simulink model "SecRwLtStHdrstUpwdDnwdHolderChk"  (R2018b)
settings: Solver=FixedStepDiscrete  StartTime=0.0  StopTime=10.0  FixedStep=0.01  RelTol=1e-3
libraries: simulink x1
settings Model: Creator=sn2xws  LastModifiedBy=sn2xws
settings Model: ModifiedHistory=|
  | 2023/11/7
  | V2.3.0 Bug555749  童锁需要停止md21 22 25 26
settings DataIOCC: SaveFormat=StructureWithTime
settings OptimizationCC: DefaultParameterBehavior=Inlined  EnhancedBackFolding=on  PassReuseOutputArgsAs=Individual arguments  ZeroExternalMemoryAtStartup=off  ZeroInternalMemoryAtStartup=off  OptimizeBlockOrder=speed  DifferentSizesBufferReuse=on  OptimizationCustomize=off
settings DebuggingCC: ParameterTunabilityLossMsg=error
settings ModelReferenceCC: ModelReferenceNumInstancesAllowed=Single
settings SFSimCC: MATLABDynamicMemAlloc=off
settings RTWCC: SystemTargetFile=autosar.tlc  GenCodeOnly=on  TemplateMakefile=ert_default_tmf  Description=AUTOSAR  GenerateReport=on  IncludeHyperlinkInReport=on  LaunchReport=on  GenerateTraceInfo=on  GenerateTraceReport=on  GenerateTraceReportSl=on  GenerateTraceReportSf=on  GenerateTraceReportEml=on
settings CodeAppCC: ForceParamTrailComments=on  IgnoreCustomStorageClasses=off  OperatorAnnotations=on  SimulinkDataObjDesc=on  SFDataObjDesc=on  InsertBlockDesc=on
settings STFCustomTargetCC: TargetLangStandard=C99 (ISO)  MultiwordLength=256  ParMdlRefBuildCompliant=on  CompOptLevelCompliant=on  IncludeMdlTerminateFcn=off  CombineOutputUpdateFcns=on  SuppressErrorStatus=on  ERTCustomFileBanners=on  SupportNonFinite=off  SupportComplex=off  SupportContinuousTime=off  SupportNonInlinedSFcns=off  RemoveResetFunc=on  MATLABClassNameForMDSCustomization=Simulink.SoftwareTarget.ERTCustomization  AutosarCompliant=on  UseToolchainInfoCompliant=on  LookupTableObjectStructAxisOrder=2,1,3,4,...  LUTObjectStructOrderEvenSpacing=Size,Table,Breakpoints  SystemTargetFile=autosar.tlc
settings ERTTargetCC: TargetLangStandard=C99 (ISO)  ConcurrentExecutionCompliant=off  IncludeMdlTerminateFcn=off  SuppressErrorStatus=on  SupportNonFinite=off  SupportComplex=off  ModelStepFunctionPrototypeControlCompliant=off  CPPClassGenCompliant=off  AutosarCompliant=on  LookupTableObjectStructAxisOrder=2,1,3,4,...  LUTObjectStructOrderEvenSpacing=Size,Table,Breakpoints  InlinedParameterPlacement=NonHierarchical  ERTCustomFileTemplate=example_file_process.tlc  ERTFilePackagingFormat=Compact

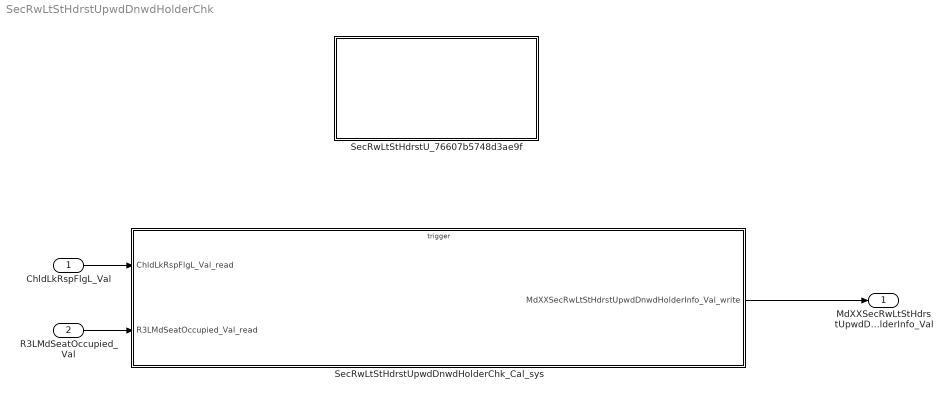
== system SecRwLtStHdrstUpwdDnwdHolderChk ==
  ChldLkRspFlgL_Val : Inport  OutDataTypeStr=boolean  PortDimensions=1
  R3LMdSeatOccupied_Val : Inport  Port=2  OutDataTypeStr=boolean  PortDimensions=1
  SecRwLtStHdrstU_76607b5748d3ae9f : Subsystem
  SecRwLtStHdrstUpwdDnwdHolderChk_Cal_sys : Subsystem
  MdXXSecRwLtStHdrstUpwdDnwdHolderInfo_Val : Outport  OutDataTypeStr=uint32  PortDimensions=1
  wires:
  ChldLkRspFlgL_Val/1 -> SecRwLtStHdrstUpwdDnwdHolderChk_Cal_sys/1(ChldLkRspFlgL_Val_read)
  R3LMdSeatOccupied_Val/1 -> SecRwLtStHdrstUpwdDnwdHolderChk_Cal_sys/2(R3LMdSeatOccupied_Val_read)
  SecRwLtStHdrstUpwdDnwdHolderChk_Cal_sys/1(MdXXSecRwLtStHdrstUpwdDnwdHolderInfo_Val_write) -> MdXXSecRwLtStHdrstUpwdDnwdHolderInfo_Val/1

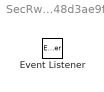
== system SecRwLtStHdrstUpwdDnwdHolderChk/SecRwLtStHdrstU_76607b5748d3ae9f ==
  Event Listener : EventListener  EventName=reset

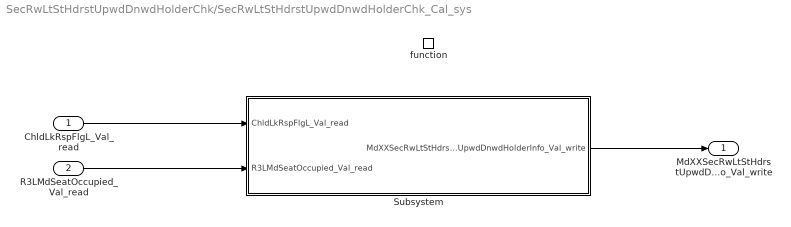
== system SecRwLtStHdrstUpwdDnwdHolderChk/SecRwLtStHdrstUpwdDnwdHolderChk_Cal_sys ==
  ChldLkRspFlgL_Val_read : Inport
  R3LMdSeatOccupied_Val_read : Inport  Port=2
  function : TriggerPort  TriggerType=function-call  IsSimulinkFunction=on  FunctionName=SecRwLtStHdrstUpwdDnwdHolderChk_Cal  VariantControl=(inherit)
  Subsystem : Subsystem
  MdXXSecRwLtStHdrstUpwdDnwdHolderInfo_Val_write : Outport
      settings: EnsureOutportIsVirtual=on
  wires:
  Subsystem/1(MdXXSecRwLtStHdrstUpwdDnwdHolderInfo_Val_write) -> MdXXSecRwLtStHdrstUpwdDnwdHolderInfo_Val_write/1
  ChldLkRspFlgL_Val_read/1 -> Subsystem/1(ChldLkRspFlgL_Val_read)
  R3LMdSeatOccupied_Val_read/1 -> Subsystem/2(R3LMdSeatOccupied_Val_read)

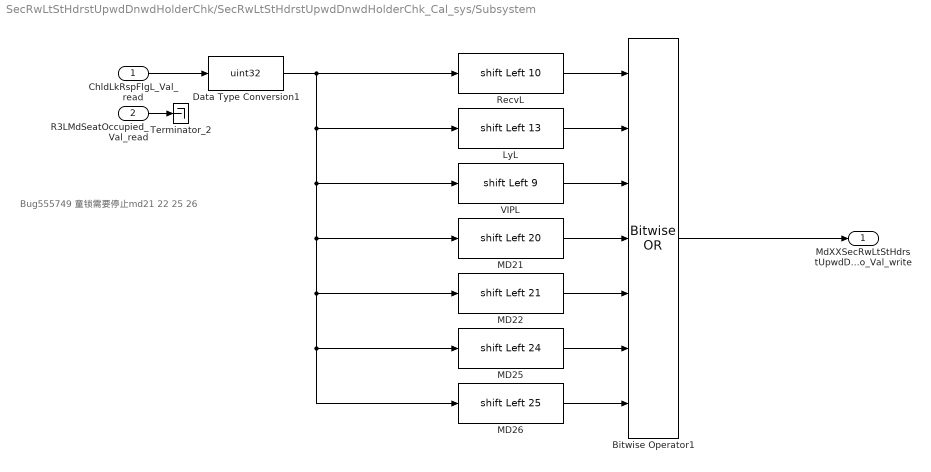
== system SecRwLtStHdrstUpwdDnwdHolderChk/SecRwLtStHdrstUpwdDnwdHolderChk_Cal_sys/Subsystem ==
  note: Bug555749 童锁需要停止md21 22 25 26
  ChldLkRspFlgL_Val_read : Inport
  R3LMdSeatOccupied_Val_read : Inport  Port=2
  Bitwise Operator1 : simulink/Logic and Bit Operations/Bitwise Operator  logicop=OR  UseBitMask=off  NumInputPorts=7  BitMask=bin2dec('11011001')  BitMaskRealWorld=Stored Integer
  Data Type Conversion1 : DataTypeConversion  OutDataTypeStr=uint32
  LyL : ArithShift  BitShiftNumber=13  BitShiftDirection=Left
  MD21 : ArithShift  BitShiftNumber=20  BitShiftDirection=Left
  MD22 : ArithShift  BitShiftNumber=21  BitShiftDirection=Left
  MD25 : ArithShift  BitShiftNumber=24  BitShiftDirection=Left
  MD26 : ArithShift  BitShiftNumber=25  BitShiftDirection=Left
  RecvL : ArithShift  BitShiftNumber=10  BitShiftDirection=Left
  Terminator_2 : Terminator
  VIPL : ArithShift  BitShiftNumber=9  BitShiftDirection=Left
  MdXXSecRwLtStHdrstUpwdDnwdHolderInfo_Val_write : Outport
      settings: EnsureOutportIsVirtual=on
  wires:
  ChldLkRspFlgL_Val_read/1 -> Data Type Conversion1/1
  R3LMdSeatOccupied_Val_read/1 -> Terminator_2/1
  Bitwise Operator1/1 -> MdXXSecRwLtStHdrstUpwdDnwdHolderInfo_Val_write/1
  VIPL/1 -> Bitwise Operator1/3
  Data Type Conversion1/1 -> RecvL/1, MD26/1, MD25/1, MD22/1, MD21/1, VIPL/1, LyL/1
  LyL/1 -> Bitwise Operator1/2
  RecvL/1 -> Bitwise Operator1/1
  MD21/1 -> Bitwise Operator1/4
  MD22/1 -> Bitwise Operator1/5
  MD25/1 -> Bitwise Operator1/6
  MD26/1 -> Bitwise Operator1/7
